simulink model "pendulo"  (Simulink 7.1)
settings: Solver=ode45  StartTime=0.0  StopTime=10.0  RelTol=1e-3
values from neighbouring files (symbols this model uses):
  B = 0.5    [pendulo.mat]
  g = 9.8    [pendulo.mat]
  L = 0.5    [pendulo.mat]
  m = 0.25    [pendulo.mat]
  M = 2    [pendulo.mat]
settings Model: Creator=ALUNO  LastModifiedBy=ALUNO

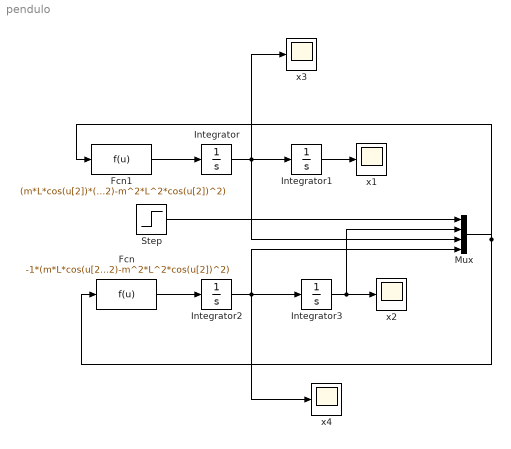
== system pendulo ==
  Fcn : Fcn  Expr=-1*(m*L*cos(u[2])*(-1*B*(u[3])+m*L*(u[4])^2*sin(u[2])+u)+(M+m)*m*g*L*sin(u[2]))/((M+m)*(4/3*m*L^2)-m^2*L^2*cos(u[2])^2)
  Fcn1 : Fcn  Expr=(m*L*cos(u[2])*(-1*B*(u[3])+m*L*(u[4])^2*sin(u[2])+u)+(M+m)*m*g*L*sin(u[2]))/((M+m)*(4/3*m*L^2)-m^2*L^2*cos(u[2])^2)
  Integrator : Integrator
  Integrator1 : Integrator
  Integrator2 : Integrator
  Integrator3 : Integrator  InitialCondition=(pi/3)
  Mux : Mux
  Step : Step  After=0  SampleTime=0
  x{1..4} (4 alike) : Scope
      x3 settings: SaveName=ScopeData2
      x4 settings: SaveName=ScopeData3
  wires:
  Fcn1/1 -> Integrator/1
  Integrator/1 -> Integrator1/1, Mux/3, x3/1
  Fcn/1 -> Integrator2/1
  Integrator2/1 -> Integrator3/1, Mux/4, x4/1
  Integrator3/1 -> x2/1, Mux/2
  Integrator1/1 -> x1/1
  Mux/1 -> Fcn/1, Fcn1/1
  Step/1 -> Mux/1
